simulink model "ATVLAB3_GABRIEL_MODELAGEM"  (R2021a)
settings: Solver=VariableStepAuto  StartTime=0.0  StopTime=10.0  RelTol=1e-3
settings Model: Creator=Aluno  LastModifiedBy=Home
settings SolverCC: AlgebraicLoopSolver=TrustRegion
settings DataIOCC: ReturnWorkspaceOutputs=off
settings DebuggingCC: SFMachineParentedDataDiag=warning  ArithmeticOperatorsInVariantConditions=warning
settings SFSimCC: SimUseLocalCustomCode=off  CustomCodeUndefinedFunction=UseInterfaceOnly
settings RTWCC: RTWUseLocalCustomCode=off

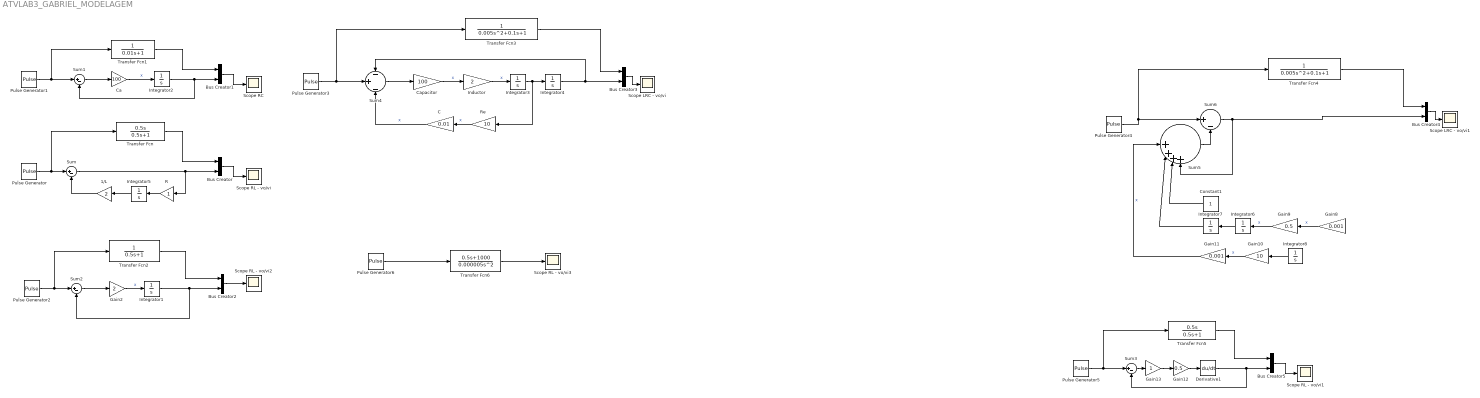
== system ATVLAB3_GABRIEL_MODELAGEM ==
  1/L : Gain  Gain=2
  Bus Creator{,1..5} (6 alike) : BusCreator  Inputs=2
  C : Gain  Gain=0.01
  Ca : Gain  Gain=100
  Capacitor : Gain  Gain=100
  Constant1 : Constant
  Derivative1 : Derivative  CoefficientInTFapproximation=1
  Gain10 : Gain  Gain=10
  Gain11 : Gain  Gain=0.001
  Gain12 : Gain  Gain=0.5
  Gain13 : Gain
  Gain2 : Gain  Gain=2
  Gain8 : Gain  Gain=0.001
  Gain9 : Gain  Gain=0.5
  Inductor : Gain  Gain=2
  Integrator{1..8} (8 alike) : Integrator
  Pulse Generator{,1..6} (7 alike) : DiscretePulseGenerator  PulseType=Time based  Amplitude=12  Period=3  PulseWidth=5
  R : Gain
  Re : Gain  Gain=10
  Scope LRC - vo/vi : Scope
  Scope LRC - vo/vi1 : Scope
  Scope RC : Scope
  Scope RL - vo/vi{,1..3} (4 alike) : Scope
  Sum{,1..3} (4 alike) : Sum  Inputs=|+-
  Sum4 : Sum  Inputs=-|+|-
  Sum5 : Sum  Inputs=|||||||+||+|+|+
  Sum6 : Sum  Inputs=||+|-
  Transfer Fcn : TransferFcn  Numerator=[0.5 0]  Denominator=[0.5 1]
  Transfer Fcn1 : TransferFcn  Denominator=[0.01 1]
  Transfer Fcn2 : TransferFcn  Denominator=[0.5 1]
  Transfer Fcn3 : TransferFcn  Denominator=[0.005 0.1 1]
  Transfer Fcn4 : TransferFcn  Denominator=[0.005 0.1 1]
  Transfer Fcn5 : TransferFcn  Numerator=[0.5 0]  Denominator=[0.5 1]
  Transfer Fcn6 : TransferFcn  Numerator=[0.5 1000]  Denominator=[0.000005 0 0]
  wires:
  Pulse Generator/1 -> Sum/1, Transfer Fcn/1
  Bus Creator/1 -> Scope RL - vo/vi/1
  Transfer Fcn/1 -> Bus Creator/1
  Integrator2/1 -> Bus Creator1/2, Sum1/2
  Transfer Fcn1/1 -> Bus Creator1/1
  Bus Creator1/1 -> Scope RC/1
  Pulse Generator1/1 -> Sum1/1, Transfer Fcn1/1
  Sum1/1 -> Ca/1
  Pulse Generator2/1 -> Sum2/1, Transfer Fcn2/1
  Sum2/1 -> Gain2/1
  Gain2/1 -> Integrator1/1  "x"
  Integrator1/1 -> Bus Creator2/2, Sum2/2
  Transfer Fcn2/1 -> Bus Creator2/1
  Ca/1 -> Integrator2/1  "x"
  Bus Creator3/1 -> Scope LRC - vo/vi/1
  Pulse Generator3/1 -> Sum4/2, Transfer Fcn3/1
  Re/1 -> C/1  "x"
  Transfer Fcn3/1 -> Bus Creator3/1
  Integrator3/1 -> Re/1, Integrator4/1
  Inductor/1 -> Integrator3/1  "x"
  Capacitor/1 -> Inductor/1  "x"
  Bus Creator4/1 -> Scope LRC - vo/vi1/1
  Transfer Fcn4/1 -> Bus Creator4/1
  Sum6/1 -> Bus Creator4/2, Sum5/4
  Constant1/1 -> Sum5/3
  Gain10/1 -> Gain11/1  "x"
  Integrator8/1 -> Gain10/1
  Pulse Generator4/1 -> Sum6/1, Transfer Fcn4/1
  Sum5/1 -> Sum6/2
  Gain11/1 -> Sum5/1  "x"
  Gain9/1 -> Integrator6/1  "x"
  Integrator7/1 -> Sum5/2
  Integrator6/1 -> Integrator7/1
  Gain8/1 -> Gain9/1  "x"
  Integrator4/1 -> Sum4/1, Bus Creator3/2
  Sum4/1 -> Capacitor/1
  C/1 -> Sum4/3  "x"
  Gain12/1 -> Derivative1/1
  Pulse Generator5/1 -> Transfer Fcn5/1, Sum3/1
  Transfer Fcn5/1 -> Bus Creator5/1
  Bus Creator5/1 -> Scope RL - vo/vi1/1
  Derivative1/1 -> Sum3/2, Bus Creator5/2
  Sum3/1 -> Gain13/1
  Gain13/1 -> Gain12/1
  Integrator5/1 -> 1/L/1
  R/1 -> Integrator5/1
  1/L/1 -> Sum/2
  Sum/1 -> R/1, Bus Creator/2
  Bus Creator2/1 -> Scope RL - vo/vi2/1
  Pulse Generator6/1 -> Transfer Fcn6/1
  Transfer Fcn6/1 -> Scope RL - vo/vi3/1
